simulink model "hospital_scenario"  (R2024b)
settings: Solver=VariableStepAuto  StartTime=0.0  StopTime=time  RelTol=1e-3
values from neighbouring files (symbols this model uses):
  m = length(data_p_arrive)    [emergency.m]
undefined symbols (not defined in the file or in its folder): entity, entitySys, get_daparture, n
settings Model: Creator=zahra  LastModifiedBy=zahra

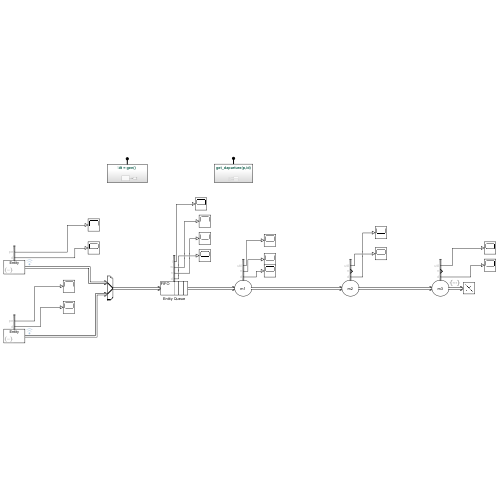
[thumbnail: Simulink's stored preview of the top-level diagram]
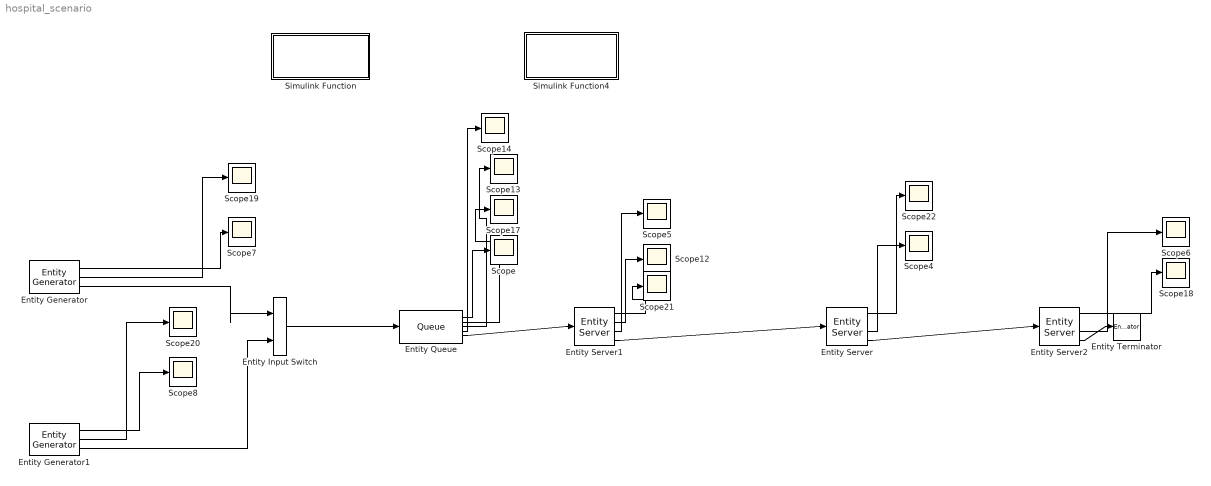
== system hospital_scenario ==
  Entity Input Switch : EntityInputSwitch  InputPortMessageModes=m,m  OutputPortMessageModes=m
  Entity Generator : EntityGenerator  OutputPortMessageModes=n,n,m  TimeSource=MATLAB action  IntergenerationTimeAction=dt=gen();  GenerateAction=|  AttributeName=stage1|stage2|stage3|type  AttributeInitialValue=1|2|0.5|1  NumberEntitiesDeparted=on  PendingEntityInBlock=on  EntityType=Structured  EntityTypeName=Entity
      | entity.stage1=exprnd(entity.stage1);
      | entity.stage2=exprnd(entity.stage2);
      | entity.stage3=exprnd(entity.stage3);
      settings: OutputPortMap=o0,o1,o3
  Entity Generator1 : EntityGenerator  OutputPortMessageModes=n,n,m  TimeSource=MATLAB action  IntergenerationTimeAction=dt=gen();  GenerateAction=|  AttributeName=stage1|stage2|stage3|type  AttributeInitialValue=0.5|2|1.5|2  NumberEntitiesDeparted=on  PendingEntityInBlock=on  EntityType=Structured  EntityTypeName=Entity
      | entity.stage1=exprnd(entity.stage1);
      | entity.stage2=exprnd(entity.stage2);
      | entity.stage3=exprnd(entity.stage3);
      settings: OutputPortMap=o0,o1,o3
  Entity Queue : Queue  InputPortMessageModes=m  OutputPortMessageModes=n,n,n,n,m  Capacity=Inf  NumberEntitiesDeparted=on  NumberEntitiesInBlock=on  AverageWait=on  AverageQueueLength=on
      settings: OutputPortMap=o0,o1,o2,o3,o5
  Entity Server : EntityServer  InputPortMessageModes=m  OutputPortMessageModes=n,n,n,m  Capacity=m2  ServiceTimeSource=Attribute  ServiceTimeAttributeName=stage2  NumberEntitiesDeparted=on  NumberEntitiesInBlock=on  Utilization=on
      settings: OutputPortMap=o0,o1,o5,o9
  Entity Server1 : EntityServer  InputPortMessageModes=m  OutputPortMessageModes=n,n,n,m  Capacity=m1  ServiceTimeSource=Attribute  ServiceTimeAttributeName=stage1  ServiceTimeAction=|  NumberEntitiesDeparted=on  NumberEntitiesInBlock=on  Utilization=on
      | % Define persistent variables
      | persistent i;
      |     
      | % Initialize the persistent variable if it's empty
      | if isempty(i)
      |    i = 1; % Start at the first index
      | end
      | 
      |  % Get stages and completion status
      | [stages, complete] = process_stage();
      | 
      | if complete==1    
      |     % Process stages if complete is 1
      |     for k = i:20
      |          dt = stages(k, 1) % Access stage data
      |                     
      |          % Increment the persistent index
      |          i = i + 1;
      |     
      |          % Exit the loop if all stages are processed
      |          if i > 20
      |               break;
      |          end
      |     end
      | end
      | dt=entity.stage1
      settings: OutputPortMap=o0,o1,o5,o9
  Entity Server2 : EntityServer  InputPortMessageModes=m  OutputPortMessageModes=n,n,n,m  Capacity=m3  ServiceTimeSource=Attribute  ServiceTimeAttributeName=stage3  ExitAction=get_daparture(entitySys.id, entity.type);  NumberEntitiesDeparted=on  NumberEntitiesInBlock=on  Utilization=on
      settings: OutputPortMap=o0,o1,o5,o9
  Entity Terminator : EntityTerminator  InputPortMessageModes=m
  Scope{,4..8,12..14,17..22} (15 alike) : Scope
  Simulink Function : Subsystem  TreatAsAtomicUnit=on
  Simulink Function4 : Subsystem  TreatAsAtomicUnit=on
  wires:
  Entity Generator1/3 -> Entity Input Switch/2
  Entity Server2/4 -> Entity Terminator/1
  Entity Server/3 -> Scope4/1
  Entity Server1/3 -> Scope5/1
  Entity Server2/3 -> Scope6/1
  Entity Queue/1 -> Scope/1
  Entity Generator/1 -> Scope7/1
  Entity Generator1/1 -> Scope8/1
  Entity Queue/5 -> Entity Server1/1
  Entity Server1/4 -> Entity Server/1
  Entity Server/4 -> Entity Server2/1
  Entity Server1/2 -> Scope12/1
  Entity Queue/3 -> Scope13/1
  Entity Queue/4 -> Scope14/1
  Entity Queue/2 -> Scope17/1
  Entity Generator/3 -> Entity Input Switch/1
  Entity Server2/1 -> Scope18/1
  Entity Generator/2 -> Scope19/1
  Entity Generator1/2 -> Scope20/1
  Entity Server1/1 -> Scope21/1
  Entity Server/1 -> Scope22/1
  Entity Input Switch/1 -> Entity Queue/1

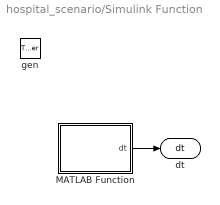
== system hospital_scenario/Simulink Function ==
  gen : TriggerPort  TriggerType=function-call  IsSimulinkFunction=on  FunctionName=gen  FunctionVisibility=scoped  VariantControl=(inherit)
  MATLAB Function : MATLAB Function  TreatAsAtomicUnit=on
  dt : ArgOut  DisableCoverage=on  ArgumentName=dt
  wires:
  MATLAB Function/1(dt) -> dt/1

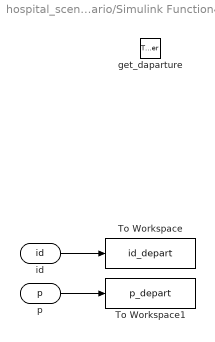
== system hospital_scenario/Simulink Function4 ==
  get_daparture : TriggerPort  TriggerType=function-call  IsSimulinkFunction=on  FunctionName=get_daparture  FunctionVisibility=scoped  VariantControl=(inherit)
  To Workspace : ToWorkspace  VariableName=id_depart  SaveFormat=Timeseries  SampleTime=-1
  To Workspace1 : ToWorkspace  VariableName=p_depart  SaveFormat=Timeseries  SampleTime=-1
  p : ArgIn  DisableCoverage=on  ArgumentName=p
  id : ArgIn  DisableCoverage=on  Port=2  ArgumentName=id
  wires:
  p/1 -> To Workspace1/1
  id/1 -> To Workspace/1

== matlab function hospital_scenario/Simulink Function/MATLAB Function ==
  data: dt output
function dt = fcn()

persistent count; % Declare a persistent variable to track entities
if isempty(count)
    count = 0; % Initialize count at the start of the simulation
end
if count < 18
    dt = 0; % Generate entities with no delay
    count = count + 1; % Increment the count
else
    dt = Inf; % Stop further entity generation
end
